simulink model "Bloque_Sensor_Airgap"  (R2022b)
settings: Solver=VariableStepAuto  StartTime=0.0  StopTime=3  RelTol=1e-3
libraries: dspstat3 x1
settings Model: Creator=aceao  LastModifiedBy=ramuj

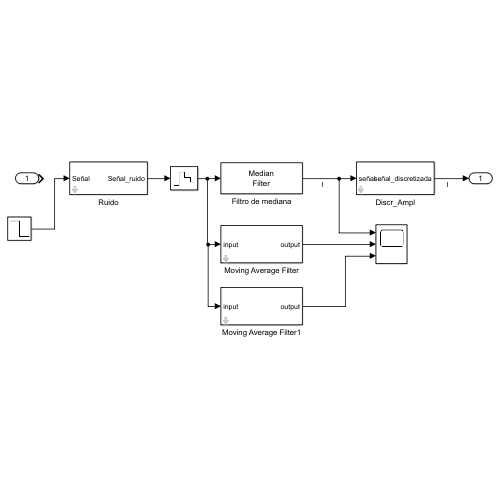
[thumbnail: Simulink's stored preview of the top-level diagram]
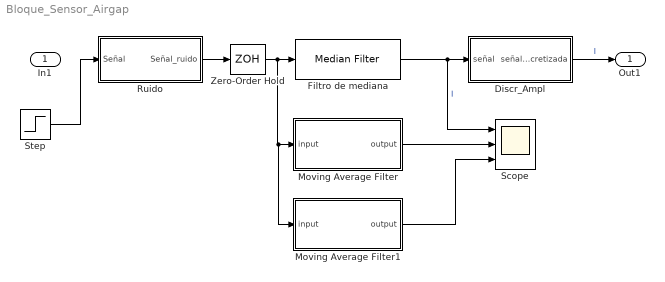
== system Bloque_Sensor_Airgap ==
  In1 : Inport
  Discr_Ampl : Subsystem  mask{N=65536, Min=4e-3, Max=20e-3}
      mask prompts: N "Valores distintos (N)"; Min "Valor mínimo"; Max "Valor máximo"
      mask DialogControl DescGroupVar Prompt: Discretizacion_Amplitud
      mask DialogControl DescTextVar Prompt: Discretización en amplitud
  Filtro de mediana : dspstat3/Median Filter  WindowLength=150  SimulateUsing=Interpreted execution
      settings: LibrarySourceBlock=|
      | dspfdesign/Median
      | Filter
  Moving Average Filter : Subsystem  mask{M=15, fs=-1}
      mask prompts: M "Orden del filtro (M)"; fs "Frecuencia de muestreo (fs)"
  Moving Average Filter1 : Subsystem  mask{M=5, fs=-1}
      mask prompts: M "Orden del filtro (M)"; fs "Frecuencia de muestreo (fs)"
  Ruido : Subsystem  mask{M=0, V=5e-6, T=0.001}
      mask prompts: M "Media"; V "Varianza"; T "Periodo"
      mask DialogControl Ruido Prompt: Ruido
      mask DialogControl DescTextVar Prompt: Añade ruido gaussiano
  Scope : Scope  NumInputPorts=3
  Step : Step  Before=0.225  After=0.185  SampleTime=0
  Zero-Order Hold : ZeroOrderHold  SampleTime=0.001
  Out1 : Outport
  wires:
  Ruido/1(Señal_ruido) -> Zero-Order Hold/1
  Zero-Order Hold/1 -> Moving Average Filter1/1(input), Moving Average Filter/1(input), Filtro de mediana/1
  Filtro de mediana/1 -> Scope/1, Discr_Ampl/1(señal)  "I"
  Discr_Ampl/1(señal_discretizada) -> Out1/1  "I"
  Moving Average Filter/1(output) -> Scope/2
  Step/1 -> Ruido/1(Señal)
  Moving Average Filter1/1(output) -> Scope/3

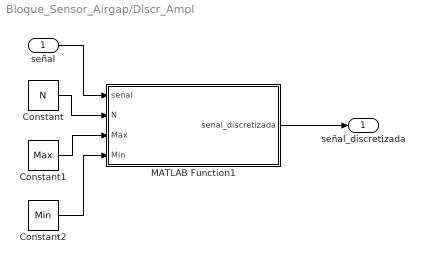
== system Bloque_Sensor_Airgap/Discr_Ampl ==
  señal : Inport
  Constant : Constant  Value=N
  Constant1 : Constant  Value=Max
  Constant2 : Constant  Value=Min
  MATLAB Function1 : MATLAB Function  TreatAsAtomicUnit=on
  señal_discretizada : Outport
  wires:
  MATLAB Function1/1(senal_discretizada) -> señal_discretizada/1
  señal/1 -> MATLAB Function1/1(senal)
  Constant1/1 -> MATLAB Function1/3(Max)
  Constant/1 -> MATLAB Function1/2(N)
  Constant2/1 -> MATLAB Function1/4(Min)

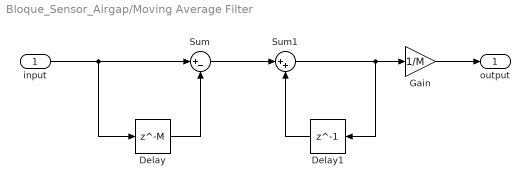
== system Bloque_Sensor_Airgap/Moving Average Filter ==
  input : Inport
  Delay : Delay  DelayLength=M  SampleTime=fs
  Delay1 : Delay  DelayLength=1  SampleTime=fs
  Gain : Gain  Gain=1/M
  Sum : Sum  Inputs=|+-
  Sum1 : Sum  Inputs=|++
  output : Outport
  wires:
  input/1 -> Delay/1, Sum/1
  Delay/1 -> Sum/2
  Sum/1 -> Sum1/1
  Sum1/1 -> Delay1/1, Gain/1
  Delay1/1 -> Sum1/2
  Gain/1 -> output/1

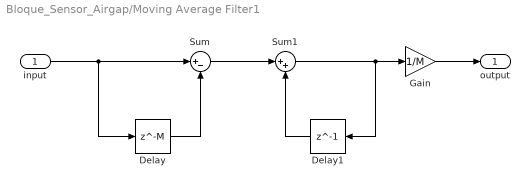
== system Bloque_Sensor_Airgap/Moving Average Filter1 ==
  input : Inport
  Delay : Delay  DelayLength=M  SampleTime=fs
  Delay1 : Delay  DelayLength=1  SampleTime=fs
  Gain : Gain  Gain=1/M
  Sum : Sum  Inputs=|+-
  Sum1 : Sum  Inputs=|++
  output : Outport
  wires:
  input/1 -> Delay/1, Sum/1
  Delay/1 -> Sum/2
  Sum/1 -> Sum1/1
  Sum1/1 -> Delay1/1, Gain/1
  Delay1/1 -> Sum1/2
  Gain/1 -> output/1

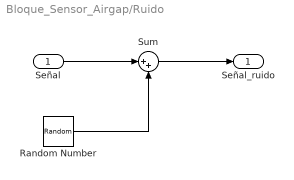
== system Bloque_Sensor_Airgap/Ruido ==
  Señal : Inport
  Random Number : RandomNumber  Mean=M  Variance=V  Seed=2  SampleTime=T
  Sum : Sum  Inputs=|++
  Señal_ruido : Outport
  wires:
  Random Number/1 -> Sum/2
  Señal/1 -> Sum/1
  Sum/1 -> Señal_ruido/1

== matlab function Bloque_Sensor_Airgap/Discr_Ampl/MATLAB Function1 ==
  data: senal input; senal_discretizada output; N input; Max input; Min input
function senal_discretizada  = fcn(senal,N,Max,Min)

if(senal>Max)
    senal_discretizada=Max;
    return
elseif(senal<Min)
    senal_discretizada=Min;
    return
end

valor_escalon=(Max-Min)/(N-1);
i=Min;
 while(i<Max)
    if(i+valor_escalon/2>senal)
        senal_discretizada=i;
        return
    end
    i=i+valor_escalon;
end

      senal_discretizada=Max;
end
